simulink model "SF102A_MotCtrlPrmEstimn"  (R2013b)
settings: Solver=FixedStepDiscrete  StartTime=0.0  StopTime=1  FixedStep=0.002  RelTol=1e-3
values from neighbouring files (symbols this model uses):
  MotCtrlPrmEstimnFetRNom = DataDict.Calibration    [SF102A_MotCtrlPrmEstimn_DataDict.m]
  MotCtrlPrmEstimnFetThermCoeff = DataDict.Calibration    [SF102A_MotCtrlPrmEstimn_DataDict.m]
  MotCtrlPrmEstimnMagThermCoeff = DataDict.Calibration    [SF102A_MotCtrlPrmEstimn_DataDict.m]
  MotCtrlPrmEstimnMotBackEmfConNom = DataDict.Calibration    [SF102A_MotCtrlPrmEstimn_DataDict.m]
  MotCtrlPrmEstimnMotBackEmfConSatnScaIvtrLoaMtgtn = DataDict.Calibration    [SF102A_MotCtrlPrmEstimn_DataDict.m]
  MotCtrlPrmEstimnMotInduDaxIvtrLoaMtgtn = DataDict.Calibration    [SF102A_MotCtrlPrmEstimn_DataDict.m]
  MotCtrlPrmEstimnMotInduDaxNom = DataDict.Calibration    [SF102A_MotCtrlPrmEstimn_DataDict.m]
  MotCtrlPrmEstimnMotInduQaxIvtrLoaMtgtn = DataDict.Calibration    [SF102A_MotCtrlPrmEstimn_DataDict.m]
  MotCtrlPrmEstimnMotInduQaxNom = DataDict.Calibration    [SF102A_MotCtrlPrmEstimn_DataDict.m]
  MotCtrlPrmEstimnMotRNom = DataDict.Calibration    [SF102A_MotCtrlPrmEstimn_DataDict.m]
  MotCtrlPrmEstimnMotWidgThermCoeff = DataDict.Calibration    [SF102A_MotCtrlPrmEstimn_DataDict.m]
  MotCtrlPrmEstimnTNom = DataDict.Calibration    [SF102A_MotCtrlPrmEstimn_DataDict.m]
libraries: NxtrLim x12, NxtrNvM x3, FixdToFloat x3, FloatToFixd x2, BilnrIntrpnCmnX x2, simulink x1, LnrIntrpn x1
(part 1 of 2)
settings Model: RequirementInfo="{}  %GIDa_d6e16671_0310_450c_8832_003ae547a212"  Creator=qzwc4r  LastModifiedBy=XZ3VZ1
settings DataIOCC: LimitDataPoints=off  SaveFormat=Structure  ReturnWorkspaceOutputs=on
settings OptimizationCC: BlockReduction=off  InlineParams=on  ZeroExternalMemoryAtStartup=off  ZeroInternalMemoryAtStartup=off  OptimizeModelRefInitCode=on  LifeSpan=1
settings DebuggingCC: SignalInfNanChecking=error  SignalRangeChecking=warning  UnderspecifiedInitializationDetection=Simplified  SolverPrmCheckMsg=error  InheritedTsInSrcMsg=error  DiscreteInheritContinuousMsg=error  MultiTaskRateTransMsg=warning  SingleTaskRateTransMsg=warning  TasksWithSamePriorityMsg=error  SigSpecEnsureSampleTimeMsg=error  CheckMatrixSingularityMsg=error  IntegerOverflowMsg=error  ParameterUnderflowMsg=error  ParameterPrecisionLossMsg=error  ParameterTunabilityLossMsg=error  FixptConstUnderflowMsg=warning  FixptConstOverflowMsg=warning  VectorMatrixConversionMsg=error  SignalLabelMismatchMsg=error  UnconnectedInputMsg=error  UnconnectedOutputMsg=error  UnconnectedLineMsg=error  SFcnCompatibilityMsg=error  UniqueDataStoreMsg=warning  BusObjectLabelMismatch=error  RootOutportRequireBusObject=error  AssertControl=DisableAll  ModelReferenceIOMsg=error  ModelReferenceVersionMismatchMessage=warning  ModelReferenceIOMismatchMessage=error  ModelReferenceCSMismatchMessage=warning  ModelReferenceDataLoggingMessage=error  StateNameClashWarn=warning  StrictBusMsg=ErrorOnBusTreatedAsVector  NonBusSignalsTreatedAsBus=error  SFUnexpectedBacktrackingDiag=error  SFInvalidInputDataAccessInChartInitDiag=error  SFNoUnconditionalDefaultTransitionDiag=error  SFTransitionOutsideNaturalParentDiag=error  SFUnconditionalTransitionShadowingDiag=error  SFUndirectedBroadcastEventsDiag=error
settings ModelReferenceCC: ModelReferenceNumInstancesAllowed=Single
settings RTWCC: SystemTargetFile=autosar.tlc  GenCodeOnly=on  TemplateMakefile=ert_default_tmf  Description=AUTOSAR  GenerateReport=on  ProcessScript=autosar_make_rtw_hook  LaunchReport=on
settings CodeAppCC: GenerateComments=off  IgnoreCustomStorageClasses=off  CustomSymbolStrType=$N$R$M  CustomSymbolStrBlkIO=$N$M  SimulinkBlockComments=off
settings STFCustomTargetCC: ParMdlRefBuildCompliant=on  CompOptLevelCompliant=on  IncludeMdlTerminateFcn=off  CombineOutputUpdateFcns=on  SuppressErrorStatus=on  ERTFirstTimeCompliant=on  ERTCustomFileBanners=on  SupportNonFinite=off  SupportComplex=off  SupportContinuousTime=off  SupportNonInlinedSFcns=off  MATLABClassNameForMDSCustomization=Simulink.SoftwareTarget.ERTCustomization  AutosarCompliant=on  GRTInterface=off  SystemTargetFile=autosar.tlc
settings ERTTargetCC: CodeReplacementLibrary=ANSI_C  ConcurrentExecutionCompliant=off  IncludeMdlTerminateFcn=off  SuppressErrorStatus=on  SupportNonFinite=off  SupportComplex=off  ModelStepFunctionPrototypeControlCompliant=off  CPPClassGenCompliant=off  AutosarCompliant=on  InlinedParameterPlacement=NonHierarchical  ERTCustomFileTemplate=example_file_process.tlc  EnableUserReplacementTypes=on

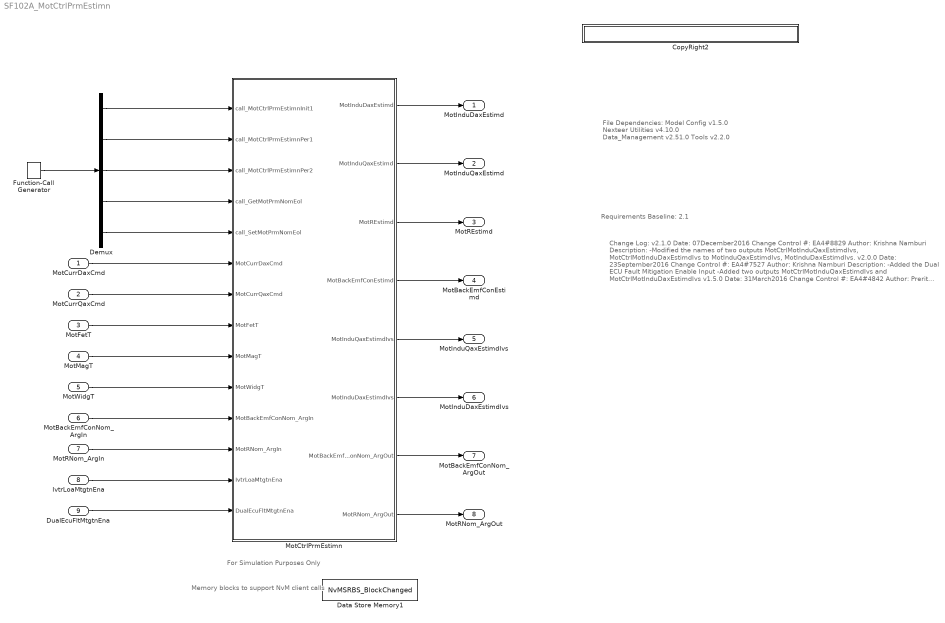
== system SF102A_MotCtrlPrmEstimn ==
  note: Memory blocks to support NvM client calls
  note: File Dependencies:
      |
      | Model Config v1.5.0
      | Nexteer Utilities v4.10.0
      | Data_Management v2.51.0
      | Tools v2.2.0
  note: Requirements Baseline: 2.1
  note: Change Log:
      |
      | v2.1.0
      | Date: 07December2016
      | Change Control #: EA4#8829
      | Author: Krishna Namburi
      | Description:
      | -Modified the names of two outputs MotCtrlMotInduQaxEstimdIvs, MotCtrlMotInduDaxEstimdIvs to
      | MotInduQaxEstimdIvs, MotInduDaxEstimdIvs.
      |
      | v2.0.0
      | Date: 23September2016
      | Change Control #: EA4#7527
      | Author: Krishna Namburi
      | Description:
      | -Added the Dual ECU Fault Mitigation Enable Input
      | -Added two outputs MotCtrlMotInduQaxEstimdIvs and MotCtrlMotInduDaxEstimdIvs
      |
      | v1.5.0
      | Date: 31March2016
      | Change Control #: EA4#4842
      | Author: Prerit Pramod
      | Description:
      | - Modified Ke saturation calculations during single inverter operation using an equation
      | - Included logic for using different nominal inductance values during single and dual inverter operation modes
      | - Added the Inverter Loss of Assist Mitigation Enable flag as a new input
      |
      | v1.4.0
      | Date: 30October2015
      | Change Control #: EA4#2393
      | Author: Fei Yuan
      | Description:
      | - Transpose the 2D table (MotCtrlPrmEstimnMotInduDaxSatnScaY, MotCtrlPrmEstimnMotInduQaxSatnScaY) to
      |    fix the dimension problem.
      | - Add a saturation block to limit the "Ke_Estimn" output from "Moto_Ke_Estimn" block.
      |
      |
      | v1.3.0
      | Date:  20August2015
      | Change Control #: EA4#1360
      | Author:  Price Lefler
      | Description:
      | - Update to the EngDT of  MotPrmNom to MotPrmNomEolRec3.
      | - Changed the Return type for the Server Runnables from 'Standard' to 'None'.
      | - Added call to SetRamBlockStatus when cal values are used to correct for corrupted NVM.
      | - TuningOwner property for calibrations were updated to comply with new allowed values.
      |
      |
      | v1.2.0
      | Date:  15July2015
      | Change Control #: EA4#1114
      | Author:  Kevin Derry
      | Description:
      | - Init runnable now overwrites PIM with cal values when NVM is corrupted.
      | - cal MotInduDaxSatnSclFacY changed to MotInduDaxSatnScaY.
      | - cal MotCtrlPrmEstimnMotInduQaxSatnSclFacY changed to MotCtrlPrmEstimnMotInduQaxSatnScaY.
      | - dMotCtrlPrmEstimnCtrlREstPreLim changed to dMotCtrlPrmEstimnCtrlrREstimdPreLim
      | - dMotCtrlPrmEstimnFetRFfEst changed to dMotCtrlPrmEstimnFetRFfEstimd
      | - dMotCtrlPrmEstimnMotBackEmfConEstPreLim changed to dMotCtrlPrmEstimnMotBackEmfConEstimdPreLim
      | - dMotCtrlPrmEstimnMotBackEmfConEstSatnSca changed to dMotCtrlPrmEstimnMotBackEmfConEstimdSatnSca
      | - dMotCtrlPrmEstimnMotInduEstPreLimDax changed to dMotCtrlPrmEstimnMotInduEstimdPreLimDax
      | - dMotCtrlPrmEstimnMotInduEstPreLimQax changed to dMotCtrlPrmEstimnMotInduEstimdPreLimQax
      | - dMotCtrlPrmEstimnMotInduEstSatnScaDax changed to dMotCtrlPrmEstimnMotInduEstimdSatnScaDax
      | - dMotCtrlPrmEstimnMotInduEstSatnScaQax changed to dMotCtrlPrmEstimnMotInduEstimdSatnScaQax
      | - dMotCtrlPrmEstimnMotRFfEst changed to dMotCtrlPrmEstimnMotRFfEstimd
      |
      |
      | v1.1.0
      | Date: 19June2015
      | Change Control #: EA4#255
      | DRW: Kevin Derry
      | Description:
      | - 'MotCtrlPrmEstimnInit' renamed 'MotCtrlPrmEstimnInit1' in model and dictionary.
      | - Units changed from VoltPerRadPerSec to VoltPerMotRadPerSec.
      | - MotCtrlPrmEstimnMotCurrQaxInduSatnX.EngMax was 250, now 200.
      | - 'MotKeNom' changed to 'MotBackEmfConNom'.
      | - Reduced number of decimal places in several calibration .EngVal values.
      | - Several display variables renamed for Autosar compliance.
      | - All dictionary entries related to FET resistance given range 0 to 0.1 Ohm.
      | - All dictionary entries related to motor or mot circut given range .005 to .12565.
      |
      |
      | v1.0.0
      | Date: 09June2015
      | Change Control #: EA4#255
      | DRW: P. Lefler
      | Description:
      | - Initial Release
  note: For Simulation Purposes Only
  MotCurrDaxCmd : Inport
  MotCurrQaxCmd : Inport  Port=2
  MotFetT : Inport  Port=3
  MotMagT : Inport  Port=4
  MotWidgT : Inport  Port=5
  MotBackEmfConNom_ArgIn : Inport  Port=6
  MotRNom_ArgIn : Inport  Port=7
  IvtrLoaMtgtnEna : Inport  Port=8
  DualEcuFltMtgtnEna : Inport  Port=9
  CopyRight2 : Subsystem  Description=|  mask(Copyright Information){none=on}
      | Copyright info block.                                               
      |                                                                     
      | Place copyright information at the top of every subsystem in design.
      mask prompts: none "No parameters"
      mask help: Place copyright information at the top of every subsystem in design.
      mask Display:
      | NxtrConf = 'Nexteer Confidential';
      | 
      | sys = bdroot; %handle for the current model ("system")
      | first = get_param(sys,'Created');
      | if(isempty(first))
      |     first = datestr(now,'yyyy');
      | else
      |     first = first(end-3:end);  %year is last four digits
      | end
      | 
      | last = get_param(sys,'LastModifiedDate');
      | if isempty(last)
      |     last = datestr(now,'yyyy');
      | else
      |     last = last(end-3:end);
      | end
      | 
      | if strcmp(first,last)
      |     fprintf('%s -- Copyright %s Nexteer',NxtrConf,first)
      | else
      |     fprintf('%s -- %s%s- %s Nexteer',NxtrConf,char(169),first,last)
      | end
  Data Store Memory1 : DataStoreMemory  DataStoreName=NvMSRBS_BlockChanged  ReadBeforeWriteMsg=warning  WriteAfterWriteMsg=warning  WriteAfterReadMsg=warning
  Demux : Demux  Outputs=5
  Function-Call Generator : simulink/Ports & Subsystems/Function-Call Generator  sample_time=0.002  numberOfIterations=1
  MotCtrlPrmEstimn : Subsystem
      settings: AttributesFormatString=%<Tag>
  MotInduDaxEstimd : Outport
  MotInduQaxEstimd : Outport  Port=2
  MotREstimd : Outport  Port=3
  MotBackEmfConEstimd : Outport  Port=4
  MotInduQaxEstimdIvs : Outport  Port=5
  MotInduDaxEstimdIvs : Outport  Port=6
  MotBackEmfConNom_ArgOut : Outport  Port=7
  MotRNom_ArgOut : Outport  Port=8
  wires:
  Demux/1 -> MotCtrlPrmEstimn/1(call_MotCtrlPrmEstimnInit1)
  Demux/2 -> MotCtrlPrmEstimn/2(call_MotCtrlPrmEstimnPer1)
  Demux/3 -> MotCtrlPrmEstimn/3(call_MotCtrlPrmEstimnPer2)
  Demux/4 -> MotCtrlPrmEstimn/4(call_GetMotPrmNomEol)
  Demux/5 -> MotCtrlPrmEstimn/5(call_SetMotPrmNomEol)
  MotCurrDaxCmd/1 -> MotCtrlPrmEstimn/6(MotCurrDaxCmd)
  MotCurrQaxCmd/1 -> MotCtrlPrmEstimn/7(MotCurrQaxCmd)
  MotCtrlPrmEstimn/1(MotInduDaxEstimd) -> MotInduDaxEstimd/1
  MotCtrlPrmEstimn/2(MotInduQaxEstimd) -> MotInduQaxEstimd/1
  MotCtrlPrmEstimn/3(MotREstimd) -> MotREstimd/1
  MotCtrlPrmEstimn/7(MotBackEmfConNom_ArgOut) -> MotBackEmfConNom_ArgOut/1
  MotCtrlPrmEstimn/8(MotRNom_ArgOut) -> MotRNom_ArgOut/1
  MotCtrlPrmEstimn/4(MotBackEmfConEstimd) -> MotBackEmfConEstimd/1
  MotCtrlPrmEstimn/5(MotInduQaxEstimdIvs) -> MotInduQaxEstimdIvs/1
  MotCtrlPrmEstimn/6(MotInduDaxEstimdIvs) -> MotInduDaxEstimdIvs/1
  MotFetT/1 -> MotCtrlPrmEstimn/8(MotFetT)
  MotMagT/1 -> MotCtrlPrmEstimn/9(MotMagT)
  MotWidgT/1 -> MotCtrlPrmEstimn/10(MotWidgT)
  MotBackEmfConNom_ArgIn/1 -> MotCtrlPrmEstimn/11(MotBackEmfConNom_ArgIn)
  MotRNom_ArgIn/1 -> MotCtrlPrmEstimn/12(MotRNom_ArgIn)
  IvtrLoaMtgtnEna/1 -> MotCtrlPrmEstimn/13(IvtrLoaMtgtnEna)
  DualEcuFltMtgtnEna/1 -> MotCtrlPrmEstimn/14(DualEcuFltMtgtnEna)
  Function-Call Generator/1 -> Demux/1

== system SF102A_MotCtrlPrmEstimn/CopyRight2 ==

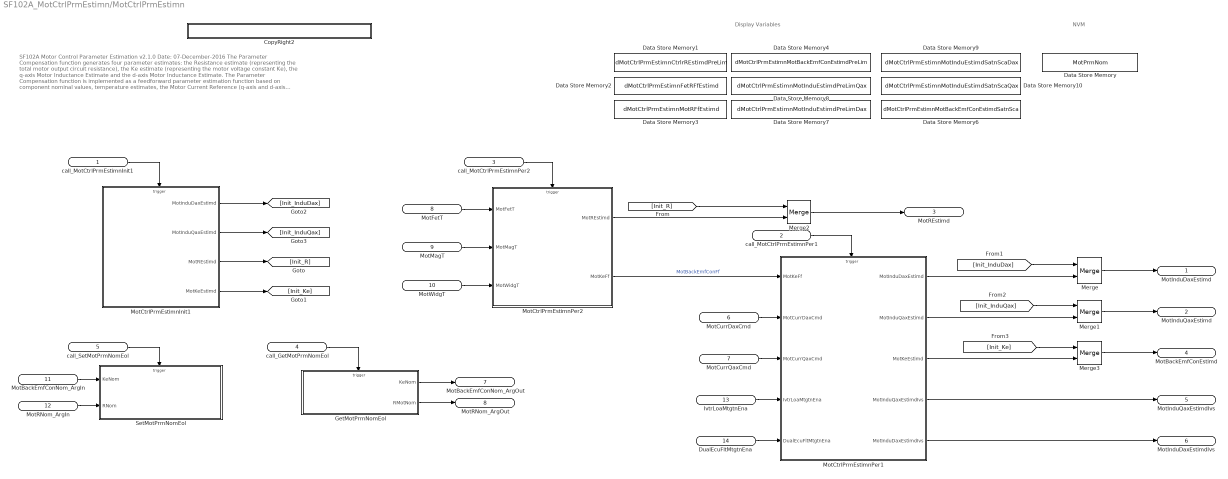
== system SF102A_MotCtrlPrmEstimn/MotCtrlPrmEstimn ==
  note: Display Variables
  note: NVM
  note: SF102A  Motor Control Parameter Estimation
      | v2.1.0      Date: 07-December-2016
      |
      | The Parameter Compensation function generates four parameter estimates: the Resistance estimate (representing the total motor output circuit resistance),
      | the Ke estimate (representing the motor voltage constant Ke), the q-axis Motor Inductance Estimate and the d-axis Motor Inductance Estimate. The
      | Parameter Compensation function is implemented as a feedforward parameter estimation function based on component nominal values, temperature estimates,
      | the Motor Current Reference (q-axis and d-axis components). The temperature dependent portion of the feedforward parameter estimation function updates
      | synchronously at the same rate as the fastest temperature estimate for the parameter (defined in the Temperature Estimation FDD).
      | All four estimates are limited by minimum and maximum calibratable limit values.
  call_MotCtrlPrmEstimnInit1 : Inport
  call_MotCtrlPrmEstimnPer1 : Inport  RequirementInfo="{'linktype_rmi_doors' '0000bb41 (/E-STEER Core/SubSystem Specifications/Application Functions/SF99/SF102A Motor Control Parameter Estimation)' '#SF102A_64' 'true' 'REQ:  SF102A_64' '' } %GIDa_20e234b7_6337_4616_ac07_9d9d8320cb43"  Port=2
  call_MotCtrlPrmEstimnPer2 : Inport  RequirementInfo="{'linktype_rmi_doors' '0000bb41 (/E-STEER Core/SubSystem Specifications/Application Functions/SF99/SF102A Motor Control Parameter Estimation)' '#SF102A_63' 'true' 'REQ:  SF102A_63' '' } %GIDa_60af119b_5c50_47b3_98ae_b61bbe6e8d7f"  Port=3
  call_GetMotPrmNomEol : Inport  Port=4
  call_SetMotPrmNomEol : Inport  Port=5
  MotCurrDaxCmd : Inport  RequirementInfo="{'linktype_rmi_doors' '0000bb41 (/E-STEER Core/SubSystem Specifications/Application Functions/SF99/SF102A Motor Control Parameter Estimation)' '#SF102A_27' 'true' 'REQ:  SF102A_27' '' } %GIDa_6c064bc6_329a_464e_9e0e_e87460f76db9"  Port=6
  MotCurrQaxCmd : Inport  RequirementInfo="{'linktype_rmi_doors' '0000bb41 (/E-STEER Core/SubSystem Specifications/Application Functions/SF99/SF102A Motor Control Parameter Estimation)' '#SF102A_36' 'true' 'REQ:  SF102A_36' '' } %GIDa_8fd35512_7c30_45b9_9067_b29c046f8ee2"  Port=7
  MotFetT : Inport  RequirementInfo="{'linktype_rmi_doors' '0000bb41 (/E-STEER Core/SubSystem Specifications/Application Functions/SF99/SF102A Motor Control Parameter Estimation)' '#SF102A_37' 'true' 'REQ:  SF102A_37' '' } %GIDa_2444ecfe_213a_483b_9d02_99490d5d5e1b"  Port=8
  MotMagT : Inport  RequirementInfo="{'linktype_rmi_doors' '0000bb41 (/E-STEER Core/SubSystem Specifications/Application Functions/SF99/SF102A Motor Control Parameter Estimation)' '#SF102A_38' 'true' 'REQ:  SF102A_38' '' } %GIDa_752e11ed_00ba_420a_b741_f580ce002643"  Port=9
  MotWidgT : Inport  RequirementInfo="{'linktype_rmi_doors' '0000bb41 (/E-STEER Core/SubSystem Specifications/Application Functions/SF99/SF102A Motor Control Parameter Estimation)' '#SF102A_39' 'true' 'REQ:  SF102A_39' '' } %GIDa_b784e2d6_8628_4597_a5f0_cbf889ab7d20"  Port=10
  MotBackEmfConNom_ArgIn : Inport  Port=11
  MotRNom_ArgIn : Inport  Port=12
  IvtrLoaMtgtnEna : Inport  RequirementInfo={'linktype_rmi_doors' '0000bb41 (/E-STEER Core/SubSystem Specifications/Application Functions/SF99/SF102A Motor Control Parameter Estimation)' '#SF102A_87' 'true' 'REQ:SF102A_87' '' } %GIDa_776d5883_5e09_460d_9808_eae134ca183a  Port=13
  DualEcuFltMtgtnEna : Inport  RequirementInfo="{'linktype_rmi_doors' '0000bb41 (/E-STEER Core/SubSystem Specifications/Application Functions/SF99/SF102A Motor Control Parameter Estimation)' '#SF102A_99' 'true' 'REQ:  SF102A_99' '' } %GIDa_163847b6_e6bc_4a53_9d21_d0786d95985f"  Port=14
  CopyRight2 : Subsystem  Description=|  mask(Copyright Information){none=on}
      | Copyright info block.                                               
      |                                                                     
      | Place copyright information at the top of every subsystem in design.
      mask prompts: none "No parameters"
      mask help: Place copyright information at the top of every subsystem in design.
      mask Display:
      | NxtrConf = 'Nexteer Confidential';
      | 
      | sys = bdroot; %handle for the current model ("system")
      | first = get_param(sys,'Created');
      | if(isempty(first))
      |     first = datestr(now,'yyyy');
      | else
      |     first = first(end-3:end);  %year is last four digits
      | end
      | 
      | last = get_param(sys,'LastModifiedDate');
      | if isempty(last)
      |     last = datestr(now,'yyyy');
      | else
      |     last = last(end-3:end);
      | end
      | 
      | if strcmp(first,last)
      |     fprintf('%s -- Copyright %s Nexteer',NxtrConf,first)
      | else
      |     fprintf('%s -- %s%s- %s Nexteer',NxtrConf,char(169),first,last)
      | end
  Data Store Memory : DataStoreMemory  DataStoreName=MotPrmNom  InitialValue=[]  OutDataTypeStr=Bus: MotPrmNomEolRec3  StateMustResolveToSignalObject=on
  Data Store Memory1 : DataStoreMemory  DataStoreName=dMotCtrlPrmEstimnCtrlrREstimdPreLim  ReadBeforeWriteMsg=warning  WriteAfterWriteMsg=warning  WriteAfterReadMsg=warning  StateMustResolveToSignalObject=on
  Data Store Memory10 : DataStoreMemory  DataStoreName=dMotCtrlPrmEstimnMotInduEstimdSatnScaQax  ReadBeforeWriteMsg=warning  WriteAfterWriteMsg=warning  WriteAfterReadMsg=warning  StateMustResolveToSignalObject=on
  Data Store Memory2 : DataStoreMemory  DataStoreName=dMotCtrlPrmEstimnFetRFfEstimd  ReadBeforeWriteMsg=warning  WriteAfterWriteMsg=warning  WriteAfterReadMsg=warning  StateMustResolveToSignalObject=on
  Data Store Memory3 : DataStoreMemory  DataStoreName=dMotCtrlPrmEstimnMotRFfEstimd  ReadBeforeWriteMsg=warning  WriteAfterWriteMsg=warning  WriteAfterReadMsg=warning  StateMustResolveToSignalObject=on
  Data Store Memory4 : DataStoreMemory  DataStoreName=dMotCtrlPrmEstimnMotBackEmfConEstimdPreLim  ReadBeforeWriteMsg=warning  WriteAfterWriteMsg=warning  WriteAfterReadMsg=warning  StateMustResolveToSignalObject=on
  Data Store Memory6 : DataStoreMemory  DataStoreName=dMotCtrlPrmEstimnMotBackEmfConEstimdSatnSca  ReadBeforeWriteMsg=warning  WriteAfterWriteMsg=warning  WriteAfterReadMsg=warning  StateMustResolveToSignalObject=on
  Data Store Memory7 : DataStoreMemory  DataStoreName=dMotCtrlPrmEstimnMotInduEstimdPreLimDax  ReadBeforeWriteMsg=warning  WriteAfterWriteMsg=warning  WriteAfterReadMsg=warning  StateMustResolveToSignalObject=on
  Data Store Memory8 : DataStoreMemory  DataStoreName=dMotCtrlPrmEstimnMotInduEstimdPreLimQax  ReadBeforeWriteMsg=warning  WriteAfterWriteMsg=warning  WriteAfterReadMsg=warning  StateMustResolveToSignalObject=on
  Data Store Memory9 : DataStoreMemory  DataStoreName=dMotCtrlPrmEstimnMotInduEstimdSatnScaDax  ReadBeforeWriteMsg=warning  WriteAfterWriteMsg=warning  WriteAfterReadMsg=warning  StateMustResolveToSignalObject=on
  GetMotPrmNomEol : Subsystem  RequirementInfo="{'linktype_rmi_doors' '0000bb41 (/E-STEER Core/SubSystem Specifications/Application Functions/SF99/SF102A Motor Control Parameter Estimation)' '#SF102A_83' 'true' 'REQ:  SF102A_83' '' } %GIDa_f0cff588_165e_4977_b84c_172dba9fa9e4"  TreatAsAtomicUnit=on
  Merge{,1..3} (4 alike) : Merge
  MotCtrlPrmEstimnInit1 : Subsystem  TreatAsAtomicUnit=on
  MotCtrlPrmEstimnPer1 : Subsystem  TreatAsAtomicUnit=on
  MotCtrlPrmEstimnPer2 : Subsystem  RequirementInfo="{'linktype_rmi_doors' '0000bb41 (/E-STEER Core/SubSystem Specifications/Application Functions/SF99/SF102A Motor Control Parameter Estimation)' '#SF102A_45' 'true' 'REQ:  SF102A_45' '' } %GIDa_db3129e3_aeec_4c11_8304_9e5d33f48bb7"  TreatAsAtomicUnit=on
  SetMotPrmNomEol : Subsystem  RequirementInfo="{'linktype_rmi_doors' '0000bb41 (/E-STEER Core/SubSystem Specifications/Application Functions/SF99/SF102A Motor Control Parameter Estimation)' '#SF102A_32' 'true' 'REQ:  SF102A_32' '' } %GIDa_5c1ea264_a025_437d_95d1_f9710e716a9a"  TreatAsAtomicUnit=on
  MotInduDaxEstimd : Outport  RequirementInfo="{'linktype_rmi_doors' '0000bb41 (/E-STEER Core/SubSystem Specifications/Application Functions/SF99/SF102A Motor Control Parameter Estimation)' '#SF102A_28' 'true' 'REQ:  SF102A_28' '' } %GIDa_eeb244ae_31d8_43f6_9b94_f5b6307d943c"
  MotInduQaxEstimd : Outport  RequirementInfo="{'linktype_rmi_doors' '0000bb41 (/E-STEER Core/SubSystem Specifications/Application Functions/SF99/SF102A Motor Control Parameter Estimation)' '#SF102A_40' 'true' 'REQ:  SF102A_40' '' } %GIDa_5b48e4d1_5c2a_4070_8988_463da3975ab3"  Port=2
  MotREstimd : Outport  RequirementInfo="{'linktype_rmi_doors' '0000bb41 (/E-STEER Core/SubSystem Specifications/Application Functions/SF99/SF102A Motor Control Parameter Estimation)' '#SF102A_41' 'true' 'REQ:  SF102A_41' '' } %GIDa_c57c517e_87f0_46b1_bc6a_762f4516709c"  Port=3
  MotBackEmfConEstimd : Outport  RequirementInfo="{'linktype_rmi_doors' '0000bb41 (/E-STEER Core/SubSystem Specifications/Application Functions/SF99/SF102A Motor Control Parameter Estimation)' '#SF102A_42' 'true' 'REQ:  SF102A_42' '' } %GIDa_e0caf834_4c81_4685_ad17_ba5200c06e6b"  Port=4
  MotInduQaxEstimdIvs : Outport  RequirementInfo="{'linktype_rmi_doors' '0000bb41 (/E-STEER Core/SubSystem Specifications/Application Functions/SF99/SF102A Motor Control Parameter Estimation)' '#SF102A_100' 'true' 'REQ:  SF102A_100' '' } %GIDa_b82b6142_f4f8_495b_b99d_7531b6c80e4d"  Port=5
  MotInduDaxEstimdIvs : Outport  RequirementInfo="{'linktype_rmi_doors' '0000bb41 (/E-STEER Core/SubSystem Specifications/Application Functions/SF99/SF102A Motor Control Parameter Estimation)' '#SF102A_101' 'true' 'REQ:  SF102A_101' '' } %GIDa_7e7770cc_94a5_4cc4_bf78_cf8c95f8a464"  Port=6
  MotBackEmfConNom_ArgOut : Outport  Port=7
  MotRNom_ArgOut : Outport  Port=8
  wires:
  call_MotCtrlPrmEstimnInit1/1 -> MotCtrlPrmEstimnInit1/Trigger
  call_MotCtrlPrmEstimnPer1/1 -> MotCtrlPrmEstimnPer1/Trigger
  call_MotCtrlPrmEstimnPer2/1 -> MotCtrlPrmEstimnPer2/Trigger
  call_GetMotPrmNomEol/1 -> GetMotPrmNomEol/Trigger
  call_SetMotPrmNomEol/1 -> SetMotPrmNomEol/Trigger
  MotFetT/1 -> MotCtrlPrmEstimnPer2/1(MotFetT)
  MotMagT/1 -> MotCtrlPrmEstimnPer2/2(MotMagT)
  MotWidgT/1 -> MotCtrlPrmEstimnPer2/3(MotWidgT)
  MotCurrDaxCmd/1 -> MotCtrlPrmEstimnPer1/2(MotCurrDaxCmd)
  MotCurrQaxCmd/1 -> MotCtrlPrmEstimnPer1/3(MotCurrQaxCmd)
  Merge/1 -> MotInduDaxEstimd/1
  Merge1/1 -> MotInduQaxEstimd/1
  MotCtrlPrmEstimnPer2/2(MotKeFf) -> MotCtrlPrmEstimnPer1/1(MotKeFf)  "MotBackEmfConFf"
  MotCtrlPrmEstimnPer2/1(MotREstimd) -> Merge2/2
  [Init_R] -> Merge2/1
  MotCtrlPrmEstimnInit1/4(MotKeEstimd) -> [Init_Ke]
  MotCtrlPrmEstimnInit1/1(MotInduDaxEstimd) -> [Init_InduDax]
  MotCtrlPrmEstimnInit1/2(MotInduQaxEstimd) -> [Init_InduQax]
  [Init_InduDax] -> Merge/1
  [Init_InduQax] -> Merge1/1
  Merge3/1 -> MotBackEmfConEstimd/1
  [Init_Ke] -> Merge3/1
  MotCtrlPrmEstimnPer1/1(MotInduDaxEstimd) -> Merge/2
  MotCtrlPrmEstimnPer1/2(MotInduQaxEstimd) -> Merge1/2
  MotBackEmfConNom_ArgIn/1 -> SetMotPrmNomEol/1(KeNom)
  MotRNom_ArgIn/1 -> SetMotPrmNomEol/2(RNom)
  GetMotPrmNomEol/1(KeNom) -> MotBackEmfConNom_ArgOut/1
  GetMotPrmNomEol/2(RMotNom) -> MotRNom_ArgOut/1
  IvtrLoaMtgtnEna/1 -> MotCtrlPrmEstimnPer1/4(IvtrLoaMtgtnEna)
  DualEcuFltMtgtnEna/1 -> MotCtrlPrmEstimnPer1/5(DualEcuFltMtgtnEna)
  MotCtrlPrmEstimnPer1/4(MotInduQaxEstimdIvs) -> MotInduQaxEstimdIvs/1
  MotCtrlPrmEstimnPer1/3(MotKeEstimd) -> Merge3/2
  MotCtrlPrmEstimnPer1/5(MotInduDaxEstimdIvs) -> MotInduDaxEstimdIvs/1
  Merge2/1 -> MotREstimd/1
  MotCtrlPrmEstimnInit1/3(MotREstimd) -> [Init_R]

== system SF102A_MotCtrlPrmEstimn/MotCtrlPrmEstimn/CopyRight2 ==

== system SF102A_MotCtrlPrmEstimn/MotCtrlPrmEstimn/GetMotPrmNomEol ==
  function : TriggerPort  TriggerType=function-call
  CopyRight2 : Subsystem  Description=|  mask(Copyright Information){none=on}
      | Copyright info block.                                               
      |                                                                     
      | Place copyright information at the top of every subsystem in design.
      mask prompts: none "No parameters"
      mask help: Place copyright information at the top of every subsystem in design.
      mask Display:
      | NxtrConf = 'Nexteer Confidential';
      | 
      | sys = bdroot; %handle for the current model ("system")
      | first = get_param(sys,'Created');
      | if(isempty(first))
      |     first = datestr(now,'yyyy');
      | else
      |     first = first(end-3:end);  %year is last four digits
      | end
      | 
      | last = get_param(sys,'LastModifiedDate');
      | if isempty(last)
      |     last = datestr(now,'yyyy');
      | else
      |     last = last(end-3:end);
      | end
      | 
      | if strcmp(first,last)
      |     fprintf('%s -- Copyright %s Nexteer',NxtrConf,first)
      | else
      |     fprintf('%s -- %s%s- %s Nexteer',NxtrConf,char(169),first,last)
      | end
  Data Store Read : DataStoreRead  RequirementInfo="{'linktype_rmi_doors' '0000bb41 (/E-STEER Core/SubSystem Specifications/Application Functions/SF99/SF102A Motor Control Parameter Estimation)' '#SF102A_83' 'true' 'REQ:  SF102A_83' '' } %GIDa_73ccec7f_42f6_446c_8aea_1c8af02359a6"  DataStoreName=MotPrmNom  DataStoreElements=MotPrmNom.MotBackEmfConNom#MotPrmNom.MotRNom
  KeNom : Outport  RequirementInfo="{'linktype_rmi_doors' '0000bb41 (/E-STEER Core/SubSystem Specifications/Application Functions/SF99/SF102A Motor Control Parameter Estimation)' '#SF102A_83' 'true' 'REQ:  SF102A_83' '' } %GIDa_10d8a1b7_7197_4734_aefa_616c56d7e0e8"
  RMotNom : Outport  RequirementInfo="{'linktype_rmi_doors' '0000bb41 (/E-STEER Core/SubSystem Specifications/Application Functions/SF99/SF102A Motor Control Parameter Estimation)' '#SF102A_83' 'true' 'REQ:  SF102A_83' '' } %GIDa_0a068918_4d21_4054_bb50_6e12ae10b93b"  Port=2
  wires:
  Data Store Read/1 -> KeNom/1
  Data Store Read/2 -> RMotNom/1

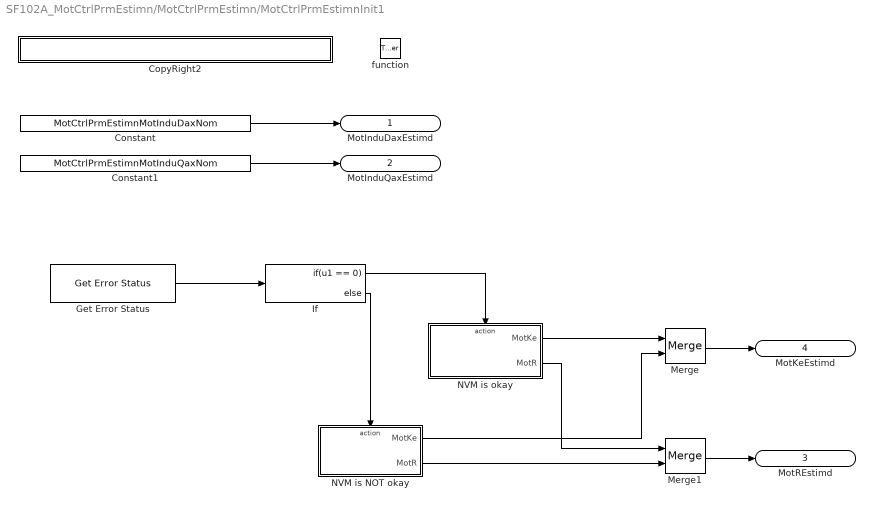
== system SF102A_MotCtrlPrmEstimn/MotCtrlPrmEstimn/MotCtrlPrmEstimnInit1 ==
  function : TriggerPort  TriggerType=function-call
  Constant : Constant  RequirementInfo="{'linktype_rmi_doors' '0000bb41 (/E-STEER Core/SubSystem Specifications/Application Functions/SF99/SF102A Motor Control Parameter Estimation)' '#SF102A_77' 'true' 'REQ:  SF102A_77' '' } %GIDa_2ed8740d_d688_4f58_ad8b_5244de0b175f"  Value=MotCtrlPrmEstimnMotInduDaxNom
  Constant1 : Constant  RequirementInfo="{'linktype_rmi_doors' '0000bb41 (/E-STEER Core/SubSystem Specifications/Application Functions/SF99/SF102A Motor Control Parameter Estimation)' '#SF102A_77' 'true' 'REQ:  SF102A_77' '' } %GIDa_136dee0c_0dc3_4114_a14a_9bbd0b7a7298"  Value=MotCtrlPrmEstimnMotInduQaxNom
  CopyRight2 : Subsystem  Description=|  mask(Copyright Information){none=on}
      | Copyright info block.                                               
      |                                                                     
      | Place copyright information at the top of every subsystem in design.
      mask prompts: none "No parameters"
      mask help: Place copyright information at the top of every subsystem in design.
      mask Display:
      | NxtrConf = 'Nexteer Confidential';
      | 
      | sys = bdroot; %handle for the current model ("system")
      | first = get_param(sys,'Created');
      | if(isempty(first))
      |     first = datestr(now,'yyyy');
      | else
      |     first = first(end-3:end);  %year is last four digits
      | end
      | 
      | last = get_param(sys,'LastModifiedDate');
      | if isempty(last)
      |     last = datestr(now,'yyyy');
      | else
      |     last = last(end-3:end);
      | end
      | 
      | if strcmp(first,last)
      |     fprintf('%s -- Copyright %s Nexteer',NxtrConf,first)
      | else
      |     fprintf('%s -- %s%s- %s Nexteer',NxtrConf,char(169),first,last)
      | end
  Get Error Status : NxtrNvM/Get Error Status  RequirementInfo="{'linktype_rmi_doors' '0000bb41 (/E-STEER Core/SubSystem Specifications/Application Functions/SF99/SF102A Motor Control Parameter Estimation)' '#SF102A_77' 'true' 'REQ:  SF102A_77' '' } %GIDa_b9a0ed49_471f_44c4_a751_d561d836d727"  FuncName=Get Error Status  NvMBlockName=MotPrmNom  VoidFuncRtn=on  ReqResPtr_DSN=NvMGES_ReqResPtr  Return_DSN=NvMGES_ReqResPtr
      settings: AttributesFormatString=%<FuncName>
  If : If  RequirementInfo="{'linktype_rmi_doors' '0000bb41 (/E-STEER Core/SubSystem Specifications/Application Functions/SF99/SF102A Motor Control Parameter Estimation)' '#SF102A_77' 'true' 'REQ:  SF102A_77' '' } %GIDa_2830ea7b_2394_48b7_a04c_a8587fbc4499"  IfExpression=u1 == 0
  Merge : Merge  RequirementInfo="{'linktype_rmi_doors' '0000bb41 (/E-STEER Core/SubSystem Specifications/Application Functions/SF99/SF102A Motor Control Parameter Estimation)' '#SF102A_77' 'true' 'REQ:  SF102A_77' '' } %GIDa_64b4aedb_cdcb_4f97_857b_3e5da3ed12b9"
  Merge1 : Merge  RequirementInfo="{'linktype_rmi_doors' '0000bb41 (/E-STEER Core/SubSystem Specifications/Application Functions/SF99/SF102A Motor Control Parameter Estimation)' '#SF102A_77' 'true' 'REQ:  SF102A_77' '' } %GIDa_7f48af0d_ffda_48b0_8cc0_6701104e3a31"
  NVM is NOT okay : Subsystem  RequirementInfo="{'linktype_rmi_doors' '0000bb41 (/E-STEER Core/SubSystem Specifications/Application Functions/SF99/SF102A Motor Control Parameter Estimation)' '#SF102A_77' 'true' 'REQ:  SF102A_77' '' } %GIDa_6f9fc078_e000_458f_ab17_1b55b17b0980"  TreatAsAtomicUnit=on
  NVM is okay : Subsystem  RequirementInfo="{'linktype_rmi_doors' '0000bb41 (/E-STEER Core/SubSystem Specifications/Application Functions/SF99/SF102A Motor Control Parameter Estimation)' '#SF102A_77' 'true' 'REQ:  SF102A_77' '' } %GIDa_5535b092_01a3_4565_b710_8e571ee4fb04"  TreatAsAtomicUnit=on
  MotInduDaxEstimd : Outport  RequirementInfo="{'linktype_rmi_doors' '0000bb41 (/E-STEER Core/SubSystem Specifications/Application Functions/SF99/SF102A Motor Control Parameter Estimation)' '#SF102A_77' 'true' 'REQ:  SF102A_77' '' } %GIDa_d015ec51_086a_4a4e_a562_d9f9a5eac8a1"
  MotInduQaxEstimd : Outport  RequirementInfo="{'linktype_rmi_doors' '0000bb41 (/E-STEER Core/SubSystem Specifications/Application Functions/SF99/SF102A Motor Control Parameter Estimation)' '#SF102A_77' 'true' 'REQ:  SF102A_77' '' } %GIDa_5abd9a3d_789a_4e6b_a8f7_2b69bc4167ae"  Port=2
  MotREstimd : Outport  RequirementInfo="{'linktype_rmi_doors' '0000bb41 (/E-STEER Core/SubSystem Specifications/Application Functions/SF99/SF102A Motor Control Parameter Estimation)' '#SF102A_77' 'true' 'REQ:  SF102A_77' '' } %GIDa_98a39883_3dc5_47a4_83d7_cd7a2b3a413e"  Port=3
  MotKeEstimd : Outport  RequirementInfo="{'linktype_rmi_doors' '0000bb41 (/E-STEER Core/SubSystem Specifications/Application Functions/SF99/SF102A Motor Control Parameter Estimation)' '#SF102A_77' 'true' 'REQ:  SF102A_77' '' } %GIDa_01db7f7f_6792_4e9a_8aa1_2ef81a2b3489"  Port=4
  wires:
  Constant/1 -> MotInduDaxEstimd/1
  Constant1/1 -> MotInduQaxEstimd/1
  Get Error Status/1 -> If/1
  If/1 -> NVM is okay/Action
  If/2 -> NVM is NOT okay/Action
  Merge/1 -> MotKeEstimd/1
  Merge1/1 -> MotREstimd/1
  NVM is okay/1(MotKe) -> Merge/1
  NVM is okay/2(MotR) -> Merge1/1
  NVM is NOT okay/1(MotKe) -> Merge/2
  NVM is NOT okay/2(MotR) -> Merge1/2

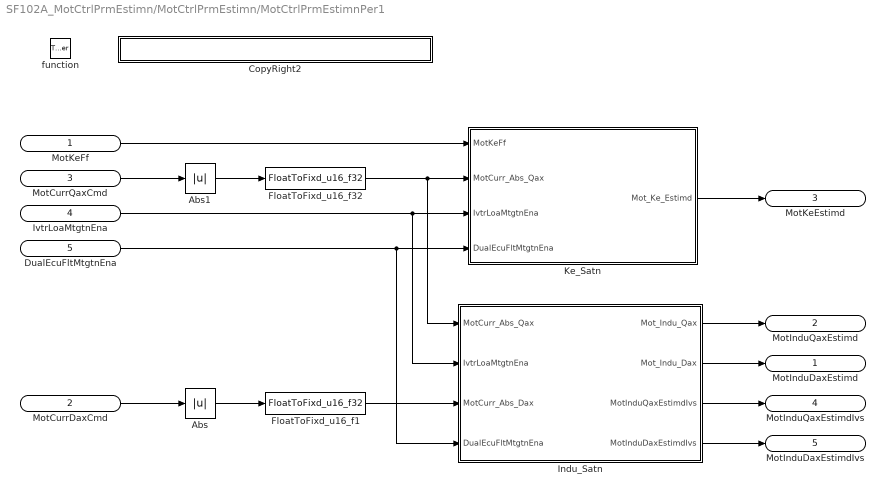
== system SF102A_MotCtrlPrmEstimn/MotCtrlPrmEstimn/MotCtrlPrmEstimnPer1 ==
  MotKeFf : Inport
  MotCurrDaxCmd : Inport  Port=2
  MotCurrQaxCmd : Inport  Port=3
  IvtrLoaMtgtnEna : Inport  RequirementInfo={} %GIDa_38641666_077e_4317_9d17_b8de0a827cde  Port=4
  DualEcuFltMtgtnEna : Inport  RequirementInfo={} %GIDa_d082cf1c_6712_4d5f_ae3b_9056d6395559  Port=5
  function : TriggerPort  TriggerType=function-call
  Abs : Abs  RequirementInfo="{'linktype_rmi_doors' '0000bb41 (/E-STEER Core/SubSystem Specifications/Application Functions/SF99/SF102A Motor Control Parameter Estimation)' '#SF102A_56' 'true' 'REQ:  SF102A_56' '' } %GIDa_12893e27_c8c0_435b_ace0_93cf443d3cdf"
  Abs1 : Abs  RequirementInfo="{'linktype_rmi_doors' '0000bb41 (/E-STEER Core/SubSystem Specifications/Application Functions/SF99/SF102A Motor Control Parameter Estimation)' '#SF102A_50' 'true' 'REQ:  SF102A_50' '' } %GIDa_24ed09ca_e3fe_445f_bde7_8f8702a4359e"
  CopyRight2 : Subsystem  Description=|  mask(Copyright Information){none=on}
      | Copyright info block.                                               
      |                                                                     
      | Place copyright information at the top of every subsystem in design.
      mask prompts: none "No parameters"
      mask help: Place copyright information at the top of every subsystem in design.
      mask Display:
      | NxtrConf = 'Nexteer Confidential';
      | 
      | sys = bdroot; %handle for the current model ("system")
      | first = get_param(sys,'Created');
      | if(isempty(first))
      |     first = datestr(now,'yyyy');
      | else
      |     first = first(end-3:end);  %year is last four digits
      | end
      | 
      | last = get_param(sys,'LastModifiedDate');
      | if isempty(last)
      |     last = datestr(now,'yyyy');
      | else
      |     last = last(end-3:end);
      | end
      | 
      | if strcmp(first,last)
      |     fprintf('%s -- Copyright %s Nexteer',NxtrConf,first)
      | else
      |     fprintf('%s -- %s%s- %s Nexteer',NxtrConf,char(169),first,last)
      | end
  FloatToFixd_u16_f1 : FloatToFixd/FloatToFixd_u16_f32  RequirementInfo="{'linktype_rmi_doors' '0000bb41 (/E-STEER Core/SubSystem Specifications/Application Functions/SF99/SF102A Motor Control Parameter Estimation)' '#SF102A_56' 'true' 'REQ:  SF102A_56' '' } %GIDa_7456eb38_78c9_430f_804d_4211f05860bb"  Param1=7
  FloatToFixd_u16_f32 : FloatToFixd/FloatToFixd_u16_f32  RequirementInfo="{'linktype_rmi_doors' '0000bb41 (/E-STEER Core/SubSystem Specifications/Application Functions/SF99/SF102A Motor Control Parameter Estimation)' '#SF102A_50' 'true' 'REQ:  SF102A_50' '' ; 'linktype_rmi_doors' '0000bb41 (/E-STEER Core/SubSystem Specifications/Application Functions/SF99/SF102A Motor Control Parameter Estimation)' '#SF102A_53' 'true' 'REQ:  SF102A_53' '' } %GIDa_b9aecf20_bfd9_42c2_a401_6d66201edd55"  Param1=7
  Indu_Satn : Subsystem
  Ke_Satn : Subsystem
  MotInduDaxEstimd : Outport
  MotInduQaxEstimd : Outport  Port=2
  MotKeEstimd : Outport  Port=3
  MotInduQaxEstimdIvs : Outport  Port=4
  MotInduDaxEstimdIvs : Outport  Port=5
  wires:
  MotKeFf/1 -> Ke_Satn/1(MotKeFf)
  MotCurrQaxCmd/1 -> Abs1/1
  MotCurrDaxCmd/1 -> Abs/1
  Abs/1 -> FloatToFixd_u16_f1/1
  Ke_Satn/1(Mot_Ke_Estimd) -> MotKeEstimd/1
  Indu_Satn/1(Mot_Indu_Qax) -> MotInduQaxEstimd/1
  Indu_Satn/2(Mot_Indu_Dax) -> MotInduDaxEstimd/1
  Abs1/1 -> FloatToFixd_u16_f32/1
  FloatToFixd_u16_f32/1 -> Indu_Satn/1(MotCurr_Abs_Qax), Ke_Satn/2(MotCurr_Abs_Qax)
  FloatToFixd_u16_f1/1 -> Indu_Satn/3(MotCurr_Abs_Dax)
  IvtrLoaMtgtnEna/1 -> Ke_Satn/3(IvtrLoaMtgtnEna), Indu_Satn/2(IvtrLoaMtgtnEna)
  DualEcuFltMtgtnEna/1 -> Indu_Satn/4(DualEcuFltMtgtnEna), Ke_Satn/4(DualEcuFltMtgtnEna)
  Indu_Satn/4(MotInduDaxEstimdIvs) -> MotInduDaxEstimdIvs/1
  Indu_Satn/3(MotInduQaxEstimdIvs) -> MotInduQaxEstimdIvs/1

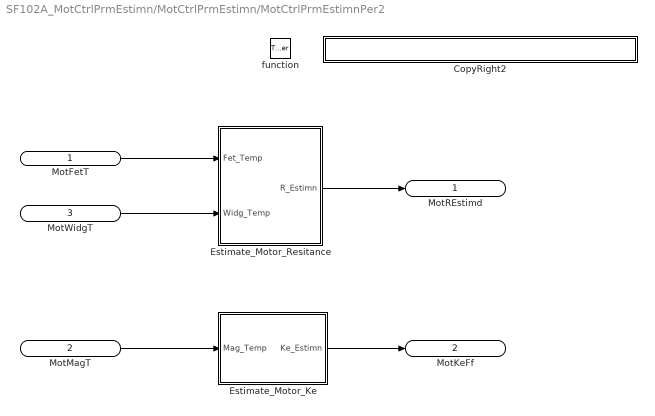
== system SF102A_MotCtrlPrmEstimn/MotCtrlPrmEstimn/MotCtrlPrmEstimnPer2 ==
  MotFetT : Inport
  MotMagT : Inport  Port=2
  MotWidgT : Inport  Port=3
  function : TriggerPort  TriggerType=function-call
  CopyRight2 : Subsystem  Description=|  mask(Copyright Information){none=on}
      | Copyright info block.                                               
      |                                                                     
      | Place copyright information at the top of every subsystem in design.
      mask prompts: none "No parameters"
      mask help: Place copyright information at the top of every subsystem in design.
      mask Display:
      | NxtrConf = 'Nexteer Confidential';
      | 
      | sys = bdroot; %handle for the current model ("system")
      | first = get_param(sys,'Created');
      | if(isempty(first))
      |     first = datestr(now,'yyyy');
      | else
      |     first = first(end-3:end);  %year is last four digits
      | end
      | 
      | last = get_param(sys,'LastModifiedDate');
      | if isempty(last)
      |     last = datestr(now,'yyyy');
      | else
      |     last = last(end-3:end);
      | end
      | 
      | if strcmp(first,last)
      |     fprintf('%s -- Copyright %s Nexteer',NxtrConf,first)
      | else
      |     fprintf('%s -- %s%s- %s Nexteer',NxtrConf,char(169),first,last)
      | end
  Estimate_Motor_Ke : Subsystem
  Estimate_Motor_Resitance : Subsystem
  MotREstimd : Outport
  MotKeFf : Outport  Port=2
  wires:
  Estimate_Motor_Resitance/1(R_Estimn) -> MotREstimd/1
  MotMagT/1 -> Estimate_Motor_Ke/1(Mag_Temp)
  MotFetT/1 -> Estimate_Motor_Resitance/1(Fet_Temp)
  MotWidgT/1 -> Estimate_Motor_Resitance/2(Widg_Temp)
  Estimate_Motor_Ke/1(Ke_Estimn) -> MotKeFf/1

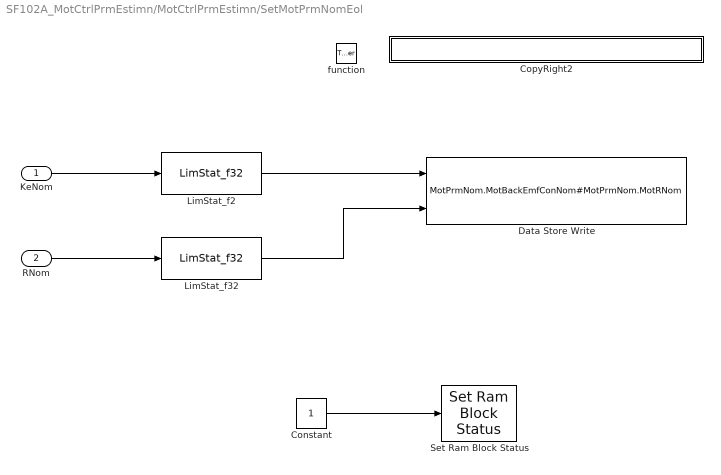
== system SF102A_MotCtrlPrmEstimn/MotCtrlPrmEstimn/SetMotPrmNomEol ==
  KeNom : Inport  RequirementInfo="{'linktype_rmi_doors' '0000bb41 (/E-STEER Core/SubSystem Specifications/Application Functions/SF99/SF102A Motor Control Parameter Estimation)' '#SF102A_81' 'true' 'REQ:  SF102A_81' '' } %GIDa_16b024e5_d763_424d_9c5c_ceb40de65f22"
  RNom : Inport  RequirementInfo="{'linktype_rmi_doors' '0000bb41 (/E-STEER Core/SubSystem Specifications/Application Functions/SF99/SF102A Motor Control Parameter Estimation)' '#SF102A_81' 'true' 'REQ:  SF102A_81' '' } %GIDa_31a623ae_eeb2_4b88_92ee_315eddd3bcf4"  Port=2
  function : TriggerPort  TriggerType=function-call
  Constant : Constant  RequirementInfo="{'linktype_rmi_doors' '0000bb41 (/E-STEER Core/SubSystem Specifications/Application Functions/SF99/SF102A Motor Control Parameter Estimation)' '#SF102A_32' 'true' 'REQ:  SF102A_32' '' } %GIDa_2d9b65ad_747a_4162_9da2_118f69d13af0"  OutDataTypeStr=double
  CopyRight2 : Subsystem  Description=|  mask(Copyright Information){none=on}
      | Copyright info block.                                               
      |                                                                     
      | Place copyright information at the top of every subsystem in design.
      mask prompts: none "No parameters"
      mask help: Place copyright information at the top of every subsystem in design.
      mask Display:
      | NxtrConf = 'Nexteer Confidential';
      | 
      | sys = bdroot; %handle for the current model ("system")
      | first = get_param(sys,'Created');
      | if(isempty(first))
      |     first = datestr(now,'yyyy');
      | else
      |     first = first(end-3:end);  %year is last four digits
      | end
      | 
      | last = get_param(sys,'LastModifiedDate');
      | if isempty(last)
      |     last = datestr(now,'yyyy');
      | else
      |     last = last(end-3:end);
      | end
      | 
      | if strcmp(first,last)
      |     fprintf('%s -- Copyright %s Nexteer',NxtrConf,first)
      | else
      |     fprintf('%s -- %s%s- %s Nexteer',NxtrConf,char(169),first,last)
      | end
  Data Store Write : DataStoreWrite  RequirementInfo="{'linktype_rmi_doors' '0000bb41 (/E-STEER Core/SubSystem Specifications/Application Functions/SF99/SF102A Motor Control Parameter Estimation)' '#SF102A_81' 'true' 'REQ:  SF102A_81' '' } %GIDa_2bb66d1f_ad08_421f_a253_ccc5f95d99be"  DataStoreName=MotPrmNom  DataStoreElements=MotPrmNom.MotBackEmfConNom#MotPrmNom.MotRNom
  LimStat_f2 : NxtrLim/LimStat_f32  RequirementInfo="{'linktype_rmi_doors' '0000bb41 (/E-STEER Core/SubSystem Specifications/Application Functions/SF99/SF102A Motor Control Parameter Estimation)' '#SF102A_58' 'true' 'REQ:  SF102A_58' '' ; 'linktype_rmi_doors' '0000bb41 (/E-STEER Core/SubSystem Specifications/Application Functions/SF99/SF102A Motor Control Parameter Estimation)' '#SF102A_77' 'true' 'REQ:  SF102A_77' '' } %GIDa_ab3b3638_61bb_4155_ad66_e96daa848660"  LoLim=MotCtrlPrmEstimnMotBackEmfConLoLim  HiLim=MotCtrlPrmEstimnMotBackEmfConHiLim
      settings: AttributesFormatString=|
      | Low Limit: %<LoLim>
      | High Limit:%<HiLim>
  LimStat_f32 : NxtrLim/LimStat_f32  RequirementInfo="{'linktype_rmi_doors' '0000bb41 (/E-STEER Core/SubSystem Specifications/Application Functions/SF99/SF102A Motor Control Parameter Estimation)' '#SF102A_59' 'true' 'REQ:  SF102A_59' '' ; 'linktype_rmi_doors' '0000bb41 (/E-STEER Core/SubSystem Specifications/Application Functions/SF99/SF102A Motor Control Parameter Estimation)' '#SF102A_77' 'true' 'REQ:  SF102A_77' '' } %GIDa_ca46b377_911f_4775_9b0a_6ab21ebbfcf8"  LoLim=MotCtrlPrmEstimnMotRLoLim  HiLim=MotCtrlPrmEstimnMotRHiLim
      settings: AttributesFormatString=|
      | Low Limit: %<LoLim>
      | High Limit:%<HiLim>
  Set Ram Block Status : NxtrNvM/Set Ram Block Status  RequirementInfo="{'linktype_rmi_doors' '0000bb41 (/E-STEER Core/SubSystem Specifications/Application Functions/SF99/SF102A Motor Control Parameter Estimation)' '#SF102A_32' 'true' 'REQ:  SF102A_32' '' } %GIDa_57b44bbf_4fc3_4519_8108_a45b6870e4c5"  FuncName=Set Ram Block Status  NvMBlockName=MotPrmNom  VoidFuncRtn=on  BlockChanged_DSN=NvMSRBS_BlockChanged  Return_DSN=NvMSRBS_Return
      settings: AttributesFormatString=%<FuncName>
  wires:
  KeNom/1 -> LimStat_f2/1
  RNom/1 -> LimStat_f32/1
  LimStat_f2/1 -> Data Store Write/1
  LimStat_f32/1 -> Data Store Write/2
  Constant/1 -> Set Ram Block Status/1

== system SF102A_MotCtrlPrmEstimn/MotCtrlPrmEstimn/GetMotPrmNomEol/CopyRight2 ==

== system SF102A_MotCtrlPrmEstimn/MotCtrlPrmEstimn/MotCtrlPrmEstimnInit1/CopyRight2 ==

== system SF102A_MotCtrlPrmEstimn/MotCtrlPrmEstimn/MotCtrlPrmEstimnInit1/NVM is NOT okay ==
  note: NVM is NOT okay. Use calibration values.
  Action Port : ActionPort  ActionType=else
  Constant : Constant  RequirementInfo={'linktype_rmi_doors' '0000bb41 (/E-STEER Core/SubSystem Specifications/Application Functions/SF99/SF102A Motor Control Parameter Estimation)' '#SF102A_77' 'true' 'REQ: SF102A_77' '' } %GIDa_61d4e754_b473_44cd_9bbf_9c47106fdc88
  Constant2 : Constant  RequirementInfo="{'linktype_rmi_doors' '0000bb41 (/E-STEER Core/SubSystem Specifications/Application Functions/SF99/SF102A Motor Control Parameter Estimation)' '#SF102A_77' 'true' 'REQ:  SF102A_77' '' } %GIDa_3c35fde2_a7f5_46de_a743_e128e2d8edbe"  Value=MotCtrlPrmEstimnMotBackEmfConNom
  Constant3 : Constant  RequirementInfo="{'linktype_rmi_doors' '0000bb41 (/E-STEER Core/SubSystem Specifications/Application Functions/SF99/SF102A Motor Control Parameter Estimation)' '#SF102A_77' 'true' 'REQ:  SF102A_77' '' } %GIDa_002c0a19_8555_4cee_abc3_a3277c475322"  Value=MotCtrlPrmEstimnMotRNom
  CopyRight2 : Subsystem  Description=|  mask(Copyright Information){none=on}
      | Copyright info block.                                               
      |                                                                     
      | Place copyright information at the top of every subsystem in design.
      mask prompts: none "No parameters"
      mask help: Place copyright information at the top of every subsystem in design.
      mask Display:
      | NxtrConf = 'Nexteer Confidential';
      | 
      | sys = bdroot; %handle for the current model ("system")
      | first = get_param(sys,'Created');
      | if(isempty(first))
      |     first = datestr(now,'yyyy');
      | else
      |     first = first(end-3:end);  %year is last four digits
      | end
      | 
      | last = get_param(sys,'LastModifiedDate');
      | if isempty(last)
      |     last = datestr(now,'yyyy');
      | else
      |     last = last(end-3:end);
      | end
      | 
      | if strcmp(first,last)
      |     fprintf('%s -- Copyright %s Nexteer',NxtrConf,first)
      | else
      |     fprintf('%s -- %s%s- %s Nexteer',NxtrConf,char(169),first,last)
      | end
  Set Ram Block Status : NxtrNvM/Set Ram Block Status  RequirementInfo={'linktype_rmi_doors' '0000bb41 (/E-STEER Core/SubSystem Specifications/Application Functions/SF99/SF102A Motor Control Parameter Estimation)' '#SF102A_77' 'true' 'REQ: SF102A_77' '' } %GIDa_b19975ea_cd1b_485a_9f40_0d38d5d95b23  FuncName=Set Ram Block Status  NvMBlockName=MotPrmNom  VoidFuncRtn=on  BlockChanged_DSN=NvMSRBS_BlockChanged  Return_DSN=NvMSRBS_Return
      settings: AttributesFormatString=%<FuncName>
  Update PIM : DataStoreWrite  RequirementInfo="{'linktype_rmi_doors' '0000bb41 (/E-STEER Core/SubSystem Specifications/Application Functions/SF99/SF102A Motor Control Parameter Estimation)' '#SF102A_77' 'true' 'REQ:  SF102A_77' '' } %GIDa_cccd2429_8851_4fe5_b66b_d5b9938c163d"  DataStoreName=MotPrmNom  DataStoreElements=MotPrmNom.MotBackEmfConNom#MotPrmNom.MotRNom
  MotKe : Outport
  MotR : Outport  Port=2
  wires:
  Constant2/1 -> Update PIM/1, MotKe/1
  Constant3/1 -> Update PIM/2, MotR/1
  Constant/1 -> Set Ram Block Status/1

== system SF102A_MotCtrlPrmEstimn/MotCtrlPrmEstimn/MotCtrlPrmEstimnInit1/NVM is okay ==
  note: NVM is okay. Use stored value
  Action Port : ActionPort  ActionType=then
  CopyRight2 : Subsystem  Description=|  mask(Copyright Information){none=on}
      | Copyright info block.                                               
      |                                                                     
      | Place copyright information at the top of every subsystem in design.
      mask prompts: none "No parameters"
      mask help: Place copyright information at the top of every subsystem in design.
      mask Display:
      | NxtrConf = 'Nexteer Confidential';
      | 
      | sys = bdroot; %handle for the current model ("system")
      | first = get_param(sys,'Created');
      | if(isempty(first))
      |     first = datestr(now,'yyyy');
      | else
      |     first = first(end-3:end);  %year is last four digits
      | end
      | 
      | last = get_param(sys,'LastModifiedDate');
      | if isempty(last)
      |     last = datestr(now,'yyyy');
      | else
      |     last = last(end-3:end);
      | end
      | 
      | if strcmp(first,last)
      |     fprintf('%s -- Copyright %s Nexteer',NxtrConf,first)
      | else
      |     fprintf('%s -- %s%s- %s Nexteer',NxtrConf,char(169),first,last)
      | end
  Data Store Read1 : DataStoreRead  RequirementInfo="{'linktype_rmi_doors' '0000bb41 (/E-STEER Core/SubSystem Specifications/Application Functions/SF99/SF102A Motor Control Parameter Estimation)' '#SF102A_77' 'true' 'REQ:  SF102A_77' '' } %GIDa_369f9c57_9e70_4cbb_ba71_6dcb2f6e50c6"  DataStoreName=MotPrmNom  DataStoreElements=MotPrmNom.MotBackEmfConNom#MotPrmNom.MotRNom
  MotKe : Outport
  MotR : Outport  Port=2
  wires:
  Data Store Read1/1 -> MotKe/1
  Data Store Read1/2 -> MotR/1

== system SF102A_MotCtrlPrmEstimn/MotCtrlPrmEstimn/MotCtrlPrmEstimnPer1/CopyRight2 ==

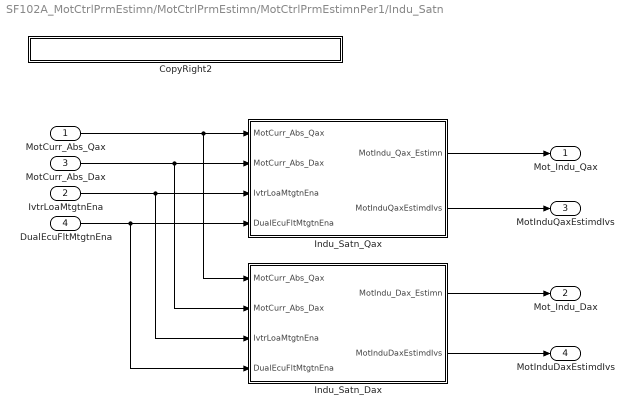
== system SF102A_MotCtrlPrmEstimn/MotCtrlPrmEstimn/MotCtrlPrmEstimnPer1/Indu_Satn ==
  MotCurr_Abs_Qax : Inport
  IvtrLoaMtgtnEna : Inport  RequirementInfo={} %GIDa_3dc5824d_f4f7_43bb_adfb_1ee1b1e01554  Port=2
  MotCurr_Abs_Dax : Inport  Port=3
  DualEcuFltMtgtnEna : Inport  RequirementInfo={} %GIDa_3082677a_43dd_4902_9d8d_6e5df8a03ced  Port=4
  CopyRight2 : Subsystem  Description=|  mask(Copyright Information){none=on}
      | Copyright info block.                                               
      |                                                                     
      | Place copyright information at the top of every subsystem in design.
      mask prompts: none "No parameters"
      mask help: Place copyright information at the top of every subsystem in design.
      mask Display:
      | NxtrConf = 'Nexteer Confidential';
      | 
      | sys = bdroot; %handle for the current model ("system")
      | first = get_param(sys,'Created');
      | if(isempty(first))
      |     first = datestr(now,'yyyy');
      | else
      |     first = first(end-3:end);  %year is last four digits
      | end
      | 
      | last = get_param(sys,'LastModifiedDate');
      | if isempty(last)
      |     last = datestr(now,'yyyy');
      | else
      |     last = last(end-3:end);
      | end
      | 
      | if strcmp(first,last)
      |     fprintf('%s -- Copyright %s Nexteer',NxtrConf,first)
      | else
      |     fprintf('%s -- %s%s- %s Nexteer',NxtrConf,char(169),first,last)
      | end
  Indu_Satn_Dax : Subsystem
  Indu_Satn_Qax : Subsystem
  Mot_Indu_Qax : Outport
  Mot_Indu_Dax : Outport  Port=2
  MotInduQaxEstimdIvs : Outport  Port=3
  MotInduDaxEstimdIvs : Outport  Port=4
  wires:
  MotCurr_Abs_Dax/1 -> Indu_Satn_Dax/2(MotCurr_Abs_Dax), Indu_Satn_Qax/2(MotCurr_Abs_Dax)
  Indu_Satn_Qax/1(MotIndu_Qax_Estimn) -> Mot_Indu_Qax/1
  Indu_Satn_Dax/1(MotIndu_Dax_Estimn) -> Mot_Indu_Dax/1
  MotCurr_Abs_Qax/1 -> Indu_Satn_Dax/1(MotCurr_Abs_Qax), Indu_Satn_Qax/1(MotCurr_Abs_Qax)
  DualEcuFltMtgtnEna/1 -> Indu_Satn_Dax/4(DualEcuFltMtgtnEna), Indu_Satn_Qax/4(DualEcuFltMtgtnEna)
  IvtrLoaMtgtnEna/1 -> Indu_Satn_Dax/3(IvtrLoaMtgtnEna), Indu_Satn_Qax/3(IvtrLoaMtgtnEna)
  Indu_Satn_Qax/2(MotInduQaxEstimdIvs) -> MotInduQaxEstimdIvs/1
  Indu_Satn_Dax/2(MotInduDaxEstimdIvs) -> MotInduDaxEstimdIvs/1
